simulink model "Intelligent_Vehicle"  (R2016a)
settings: Solver=FixedStepDiscrete  SolverMode=SingleTasking  StartTime=0.0  StopTime=350  FixedStep=1  RelTol=1e-3
libraries: simulink x1
settings Model: Creator=ihong-gyu  LastModifiedBy=Junghoon
settings DataIOCC: LimitDataPoints=on
settings OptimizationCC: DefaultParameterBehavior=Inlined  UseFloatMulNetSlope=on  InlineInvariantSignals=on  PassReuseOutputArgsAs=Individual arguments  ZeroExternalMemoryAtStartup=off  ZeroInternalMemoryAtStartup=off  NoFixptDivByZeroProtection=on  EfficientFloat2IntCast=on  OptimizeModelRefInitCode=on  LifeSpan=1
settings DebuggingCC: AllowSymbolicDim=off
settings HardwareCC: ProdBitPerPointer=32  ProdLargestAtomicFloat=None  ProdWordSize=32  ProdHWDeviceType=Infineon->TriCore
settings ModelReferenceCC: PropagateSignalLabelsOutOfModel=off
settings RTWCC: SystemTargetFile=ert.tlc  GenCodeOnly=on  TemplateMakefile=ert_default_tmf  GenerateReport=on  IncludeHyperlinkInReport=on  LaunchReport=on  GenerateTraceInfo=on  GenerateTraceReport=on  GenerateTraceReportSl=on  GenerateTraceReportSf=on  GenerateTraceReportEml=on  GenerateCodeMetricsReport=on
settings CodeAppCC: ForceParamTrailComments=on  IgnoreCustomStorageClasses=off  SimulinkDataObjDesc=on  CustomSymbolStrGlobalVar=rt$N$M  CustomSymbolStrType=$N$M  CustomSymbolStrFcn=$N$M$F  CustomSymbolStrMacro=$N$M  InsertBlockDesc=on
settings ERTTargetCC: GenerateSampleERTMain=on  IncludeMdlTerminateFcn=off  CombineSignalStateStructs=on  SupportNonFinite=off  InlinedParameterPlacement=NonHierarchical  ERTCustomFileTemplate=example_file_process.tlc  ERTFilePackagingFormat=CompactWithDataFile  PreserveExpressionOrder=on  PreserveIfCondition=on  ConvertIfToSwitch=off  SuppressUnreachableDefaultCases=off
settings ConfigurationSet: Description=SimMechanics 2G

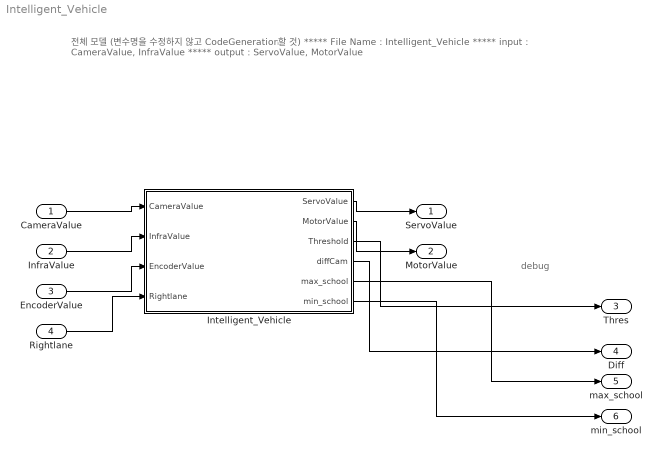
== system Intelligent_Vehicle ==
  note: debug
  note: 전체 모델
      | (변수명을 수정하지 않고 CodeGeneration할 것)
      |
      | ***** File Name : Intelligent_Vehicle
      | ***** input : CameraValue, InfraValue
      | ***** output : ServoValue, MotorValue
  CameraValue : Inport
  InfraValue : Inport  Port=2
  EncoderValue : Inport  Port=3
  Rightlane : Inport  Port=4
  "Intelligent_Vehicle " : Subsystem
      mask Display: image(imread('Images/self.jpeg'))
  ServoValue : Outport
  MotorValue : Outport  Port=2  OutDataTypeStr=int16
  Thres : Outport  Port=3
  Diff : Outport  Port=4
  max_school : Outport  Port=5
  min_school : Outport  Port=6
  wires:
  CameraValue/1 -> "Intelligent_Vehicle "/1(CameraValue)
  "Intelligent_Vehicle "/1(ServoValue) -> ServoValue/1
  "Intelligent_Vehicle "/2(MotorValue) -> MotorValue/1
  InfraValue/1 -> "Intelligent_Vehicle "/2(InfraValue)
  "Intelligent_Vehicle "/3(Threshold) -> Thres/1
  "Intelligent_Vehicle "/4(diffCam) -> Diff/1
  "Intelligent_Vehicle "/5(max_school) -> max_school/1
  "Intelligent_Vehicle "/6(min_school) -> min_school/1
  EncoderValue/1 -> "Intelligent_Vehicle "/3(EncoderValue)
  Rightlane/1 -> "Intelligent_Vehicle "/4(Rightlane)

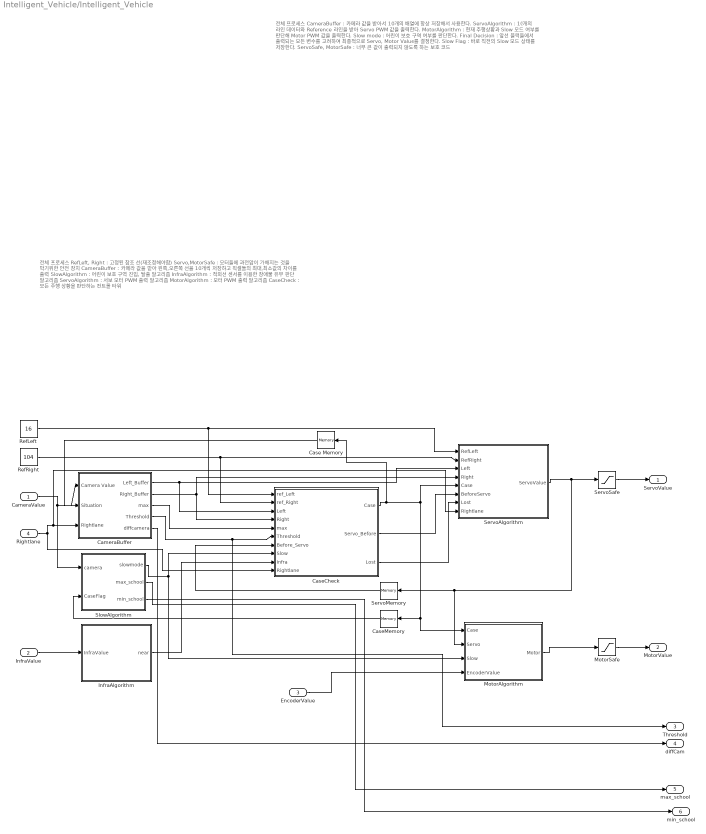
== system Intelligent_Vehicle/Intelligent_Vehicle  ==
  note: 전체 프로세스
      |
      | CameraBuffer : 카메라 값을 받아서 10개의 배열에 항상 저장해서 사용한다.
      | ServoAlgorithm : 10개의 라인 데이터와 Reference 라인을 받아 Servo PWM 값을 출력한다.
      | MotorAlgorithm : 현재 주행상황과 Slow 모드 여부를 판단해 Motor PWM 값을 출력한다.
      | Slow mode : 어린이 보호 구역 여부를 판단한다.
      | Final Decision : 앞선 블럭들에서 출력되는 모든 변수를 고려하여 최종적으로 Servo, Motor Value를 결정한다.
      | Slow Flag : 바로 직전의 Slow 모드 상태를 저장한다.
      | ServoSafe, MotorSafe : 너무 큰 값이 출력되지 않도록 하는 보호 코드
  note: 전체 프로세스
      |
      | RefLeft, Right : 고정된 참조 선(재조정해야함)
      | Servo,MotorSafe : 모터들에 과전압이 가해지는 것을 막기위한 안전 장치
      | CameraBuffer : 카메라 값을 받아 왼쪽,오른쪽 선을 10개씩 저장하고 픽셀들의 최대,최소값의 차이를 출력
      | SlowAlgorithm : 어린이 보호 구역 진입, 탈출 알고리즘
      | InfraAlgorithm : 적외선 센서를 이용한 장애물 유무 판단 알고리즘
      | ServoAlgorithm : 서보 모터 PWM 출력 알고리즘
      | MotorAlgorithm : 모터 PWM 출력 알고리즘
      | CaseCheck : 모든 주행 상황을 판단하는 컨트롤 타워
  CameraValue : Inport
  InfraValue : Inport  Port=2
  EncoderValue : Inport  Port=3
  Rightlane : Inport  Port=4
  CameraBuffer : Subsystem
      mask Display: image(imread('Images/linescan.jpg'))
  Case Memory : Memory  X0=1
  CaseCheck : MATLAB Function  TreatAsAtomicUnit=on
  CaseMemory : Memory
  InfraAlgorithm : MATLAB Function  TreatAsAtomicUnit=on
  MotorAlgorithm : Subsystem
      mask Display: image(imread('Images/dcmotor.jpeg'))
  MotorSafe : Saturate  UpperLimit=450  LowerLimit=-450
  RefLeft : Constant  Value=16  OutDataTypeStr=int16
  RefRight : Constant  Value=104  OutDataTypeStr=int16
  ServoAlgorithm : Subsystem
      mask Display: image(imread('Images/servo.jpg'))
  ServoMemory : Memory
  ServoSafe : Saturate  UpperLimit=100  LowerLimit=-100
  SlowAlgorithm : MATLAB Function  TreatAsAtomicUnit=on
  ServoValue : Outport
  MotorValue : Outport  Port=2  OutDataTypeStr=int16
  Threshold : Outport  Port=3
  diffCam : Outport  Port=4
  max_school : Outport  Port=5
  min_school : Outport  Port=6
  wires:
  CameraValue/1 -> CameraBuffer/1(Camera Value), SlowAlgorithm/1(camera)
  CaseCheck/1(Case) -> ServoAlgorithm/5(Case), MotorAlgorithm/1(Case), CaseMemory/1, Case Memory/1
  InfraValue/1 -> InfraAlgorithm/1(InfraValue)
  InfraAlgorithm/1(near) -> CaseCheck/9(Infra)
  ServoSafe/1 -> ServoValue/1
  MotorSafe/1 -> MotorValue/1
  CameraBuffer/3(max) -> CaseCheck/5(max)
  RefRight/1 -> ServoAlgorithm/2(RefRight), CaseCheck/2(ref_Right)
  RefLeft/1 -> ServoAlgorithm/1(RefLeft), CaseCheck/1(ref_Left)
  CameraBuffer/2(Right_Buffer) -> ServoAlgorithm/4(Right), CaseCheck/4(Right)
  CameraBuffer/1(Left_Buffer) -> ServoAlgorithm/3(Left), CaseCheck/3(Left)
  CaseCheck/2(Servo_Before) -> ServoAlgorithm/6(BeforeServo)
  ServoAlgorithm/1(ServoValue) -> MotorAlgorithm/2(Servo), ServoMemory/1, ServoSafe/1
  SlowAlgorithm/1(slowmode) -> CaseCheck/8(Slow), MotorAlgorithm/3(Slow)
  CaseMemory/1 -> SlowAlgorithm/2(CaseFlag)
  CaseCheck/3(Lost) -> ServoAlgorithm/7(Lost)
  ServoMemory/1 -> CaseCheck/7(Before_Servo)
  MotorAlgorithm/1(Motor) -> MotorSafe/1
  CameraBuffer/4(Threshold) -> Threshold/1, CaseCheck/6(Threshold)
  CameraBuffer/5(diffcamera) -> diffCam/1
  SlowAlgorithm/2(max_school) -> max_school/1
  SlowAlgorithm/3(min_school) -> min_school/1
  Case Memory/1 -> CameraBuffer/2(Situation)
  Rightlane/1 -> CaseCheck/10(Rightlane), ServoAlgorithm/8(Rightlane), CameraBuffer/3(Rightlane)
  EncoderValue/1 -> MotorAlgorithm/4(EncoderValue)

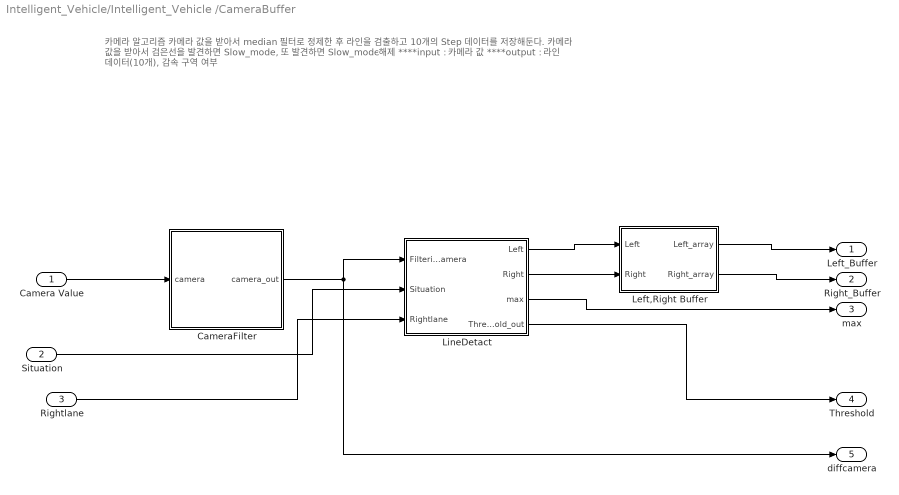
== system Intelligent_Vehicle/Intelligent_Vehicle /CameraBuffer ==
  note: 카메라 알고리즘
      |
      | 카메라 값을 받아서 median 필터로 정제한 후 라인을 검출하고 10개의 Step 데이터를 저장해둔다.
      | 카메라 값을 받아서 검은선을 발견하면 Slow_mode, 또 발견하면 Slow_mode해제
      |
      | ****input : 카메라 값
      | ****output : 라인 데이터(10개), 감속 구역 여부
  Camera Value : Inport  OutMin=[128]  OutMax=[128]  OutDataTypeStr=int16
  Situation : Inport  Port=2  OutMin=[128]  OutMax=[128]  OutDataTypeStr=int16
  Rightlane : Inport  Port=3  OutMin=[128]  OutMax=[128]  OutDataTypeStr=int16
  CameraFilter : MATLAB Function  TreatAsAtomicUnit=on
  Left,Right Buffer : MATLAB Function  TreatAsAtomicUnit=on
  LineDetact : MATLAB Function  TreatAsAtomicUnit=on
  Left_Buffer : Outport  OutMax=[10]  OutDataTypeStr=int16
  Right_Buffer : Outport  Port=2  OutMax=[10]  OutDataTypeStr=int16
  max : Outport  Port=3  OutMax=[10]  OutDataTypeStr=int16
  Threshold : Outport  Port=4  OutMax=[10]  OutDataTypeStr=int16
  diffcamera : Outport  Port=5  OutMax=[10]  OutDataTypeStr=int16
  wires:
  Left,Right Buffer/2(Right_array) -> Right_Buffer/1
  Left,Right Buffer/1(Left_array) -> Left_Buffer/1
  LineDetact/1(Left) -> Left,Right Buffer/1(Left)
  LineDetact/2(Right) -> Left,Right Buffer/2(Right)
  Camera Value/1 -> CameraFilter/1(camera)
  LineDetact/3(max) -> max/1
  CameraFilter/1(camera_out) -> diffcamera/1, LineDetact/1(Filtering_Camera)
  LineDetact/4(Threshold_out) -> Threshold/1
  Situation/1 -> LineDetact/2(Situation)
  Rightlane/1 -> LineDetact/3(Rightlane)

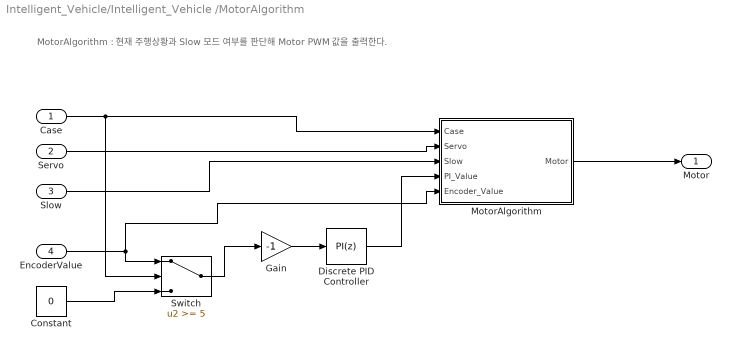
== system Intelligent_Vehicle/Intelligent_Vehicle /MotorAlgorithm ==
  note: MotorAlgorithm : 현재 주행상황과 Slow 모드 여부를 판단해 Motor PWM 값을 출력한다.
  Case : Inport  OutDataTypeStr=int16
  Servo : Inport  Port=2  OutDataTypeStr=int16
  Slow : Inport  Port=3  OutDataTypeStr=int16
  EncoderValue : Inport  Port=4  OutDataTypeStr=int16
  Constant : Constant  Value=0  OutDataTypeStr=int16
  Discrete PID Controller : simulink/Continuous/PID Controller  Controller=PI  TimeDomain=Discrete-time  SampleTime=1  IntegratorMethod=Forward Euler  FilterMethod=Forward Euler  Form=Parallel  UseFilter=on  ControllerParametersSource=internal  P=2.7  I=0.01  D=0  N=100  InitialConditionSource=internal  InitialConditionForIntegrator=0  InitialConditionForFilter=0  ExternalReset=none  ZeroCross=off  LimitOutput=on  UpperSaturationLimit=250  LowerSaturationLimit=-350  LinearizeAsGain=off  AntiWindupMode=none  Kb=1  TrackingMode=off  Kt=1  PParamMin=[]  PParamMax=[]  PParamDataTypeStr=double  IParamMin=[]  IParamMax=[]  IParamDataTypeStr=double  DParamMin=[]  DParamMax=[]  NParamMin=[]  NParamMax=[]  KbParamMin=[]  KbParamMax=[]  KtParamMin=[]  KtParamMax=[]  POutMin=[]  POutMax=[]  POutDataTypeStr=double  PGainOutDataTypeStr=double  PProdOutDataTypeStr=double  IOutMin=[]  IOutMax=[]  IOutDataTypeStr=double  IGainOutDataTypeStr=double  IProdOutDataTypeStr=double  DOutMin=[]  DOutMax=[]  NOutMin=[]  NOutMax=[]  KbOutMin=[]  KbOutMax=[]  KtOutMin=[]  KtOutMax=[]  IntegratorOutMin=[]  IntegratorOutMax=[]  IntegratorOutDataTypeStr=double  FilterOutMin=[]  FilterOutMax=[]  SumOutMin=[]  SumOutMax=[]  SumI1OutMin=[]  SumI1OutMax=[]  SumI2OutMin=[]  SumI2OutMax=[]  SumI3OutMin=[]  SumI3OutMax=[]  SumDOutMin=[]  SumDOutMax=[]  SaturationOutMin=[]  SaturationOutMax=[]  SaturationOutDataTypeStr=double  IntegratorContinuousStateAttributes=''  IntegratorStateMustResolveToSignalObject=off  IntegratorRTWStateStorageClass=Auto  FilterContinuousStateAttributes=''  FilterStateMustResolveToSignalObject=off  FilterRTWStateStorageClass=Auto  DifferentiatorICPrevScaledInput=0  DifferentiatorOutMin=[]  DifferentiatorOutMax=[]
  Gain : Gain  Gain=-1
  "MotorAlgorithm " : MATLAB Function  TreatAsAtomicUnit=on
  Switch : Switch  Threshold=5
  Motor : Outport  OutDataTypeStr=int16
  wires:
  Case/1 -> "MotorAlgorithm "/1(Case), Switch/2
  Servo/1 -> "MotorAlgorithm "/2(Servo)
  Slow/1 -> "MotorAlgorithm "/3(Slow)
  "MotorAlgorithm "/1(Motor) -> Motor/1
  Discrete PID Controller/1 -> "MotorAlgorithm "/4(PI_Value)
  Gain/1 -> Discrete PID Controller/1
  Switch/1 -> Gain/1
  Constant/1 -> Switch/3
  EncoderValue/1 -> Switch/1, "MotorAlgorithm "/5(Encoder_Value)

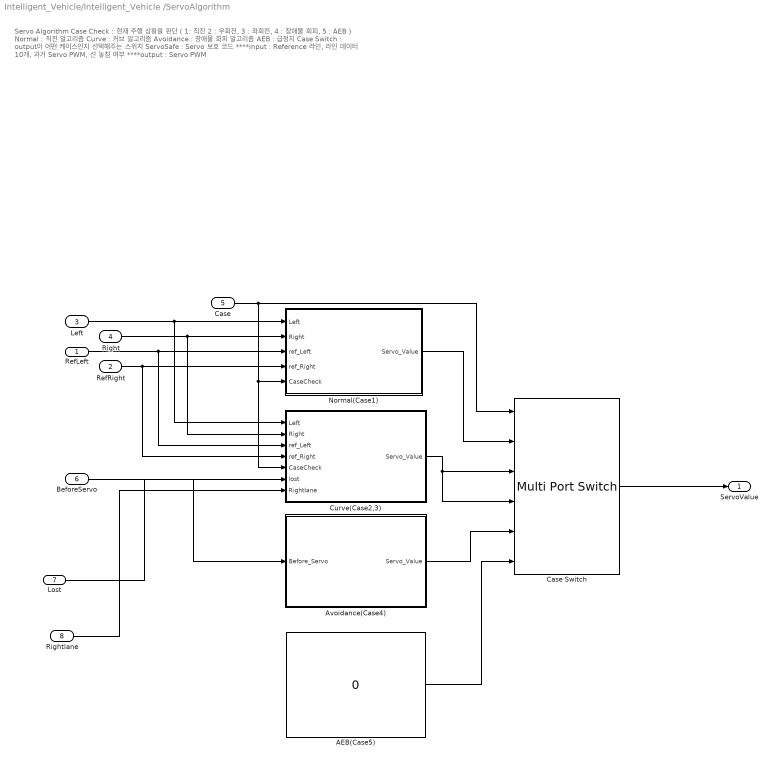
== system Intelligent_Vehicle/Intelligent_Vehicle /ServoAlgorithm ==
  note: Servo Algorithm
      |
      | Case Check : 현재 주행 상황을 판단 ( 1: 직진 2 : 우회전, 3 : 좌회전, 4 : 장애물 회피, 5 : AEB )
      | Normal : 직진 알고리즘
      | Curve : 커브 알고리즘
      | Avoidance : 장애물 회피 알고리즘
      | AEB : 급정지
      | Case Switch : output이 어떤 케이스인지 선택해주는 스위치
      | ServoSafe : Servo 보호 코드
      |
      | ****input : Reference 라인, 라인 데이터 10개, 과거 Servo PWM, 선 놓침 여부
      | ****output : Servo PWM
  RefLeft : Inport
  RefRight : Inport  Port=2
  Left : Inport  Port=3
  Right : Inport  Port=4
  Case : Inport  Port=5
  BeforeServo : Inport  Port=6
  Lost : Inport  Port=7
  Rightlane : Inport  Port=8
  AEB(Case5) : Constant  Value=0  OutDataTypeStr=int16
      mask Display: image(imread('Images/aeb.png'))
  Avoidance(Case4) : MATLAB Function  TreatAsAtomicUnit=on
  Case Switch : MultiPortSwitch  Inputs=5
      mask Display: image(imread('Images/switch.jpg'))
  Curve(Case2,3) : MATLAB Function  TreatAsAtomicUnit=on
  Normal(Case1) : MATLAB Function  TreatAsAtomicUnit=on
  ServoValue : Outport
  wires:
  Lost/1 -> Curve(Case2,3)/6(lost)
  Right/1 -> Curve(Case2,3)/2(Right), Normal(Case1)/2(Right)
  Case Switch/1 -> ServoValue/1
  RefRight/1 -> Curve(Case2,3)/4(ref_Right), Normal(Case1)/4(ref_Right)
  Curve(Case2,3)/1(Servo_Value) -> Case Switch/4, Case Switch/3
  BeforeServo/1 -> Avoidance(Case4)/1(Before_Servo)
  Normal(Case1)/1(Servo_Value) -> Case Switch/2
  Left/1 -> Curve(Case2,3)/1(Left), Normal(Case1)/1(Left)
  Case/1 -> Curve(Case2,3)/5(CaseCheck), Normal(Case1)/5(CaseCheck), Case Switch/1
  RefLeft/1 -> Curve(Case2,3)/3(ref_Left), Normal(Case1)/3(ref_Left)
  Avoidance(Case4)/1(Servo_Value) -> Case Switch/5
  AEB(Case5)/1 -> Case Switch/6
  Rightlane/1 -> Curve(Case2,3)/7(Rightlane)

== matlab function Intelligent_Vehicle/Intelligent_Vehicle /CameraBuffer/CameraFilter ==
  data: camera input int16 size=128; camera_out output int16 size=128
function camera_out= fcn(camera)

%%made by HongKyu 06.22
%%카메라 필터 모듈
%%카메라 값을 받아서 median 필터를 거친 후 차분값을 저장한다

%%전역 변수 초기화
persistent  lastpixel;
persistent  diff_camera;



if isempty(lastpixel)
    lastpixel=int16(1500);
end
if isempty(diff_camera)
    diff_camera = camera;
end



%%지역 변수 초기화
camera_out = camera;


%% 끝값들을 필터 적용(3,4개씩) 


%% 중간값들을 필터 적용 (5개씩)


%% 차분을 저장 
for i=2:128
    
    diff_camera(i)=camera(i)-lastpixel;
    camera_out(i)=diff_camera(i);
    lastpixel=camera(i-1);
end

== matlab function Intelligent_Vehicle/Intelligent_Vehicle /CameraBuffer/LineDetact ==
  data: Filtering_Camera input int16 size=128; Left output int16 size=1; Right output int16 size=1; max output; Threshold_out output; Situation input; Rightlane input
function [Left,Right,max,Threshold_out] = fcn(Filtering_Camera,Situation, Rightlane)

%%made by HongKyu 06.22
%%라인 검출 모듈
%%필터링 된 카메라 차분 값 중에서 변화의 최대값을 선으로 인식한다
%%최소값을 저장하는 이유는 SLOW 모드를 받아들일 때 사용하려 했으나 우꿍1 알고리즘을 참고하여 사용안할 예정 
%%알고리즘 by 우꿍2

%%전역 변수 초기화 
persistent maxmindiff;
persistent LPF_initcount;
persistent  array_max;
persistent  sum_max;
persistent Threshold;

if isempty(maxmindiff)
    maxmindiff = 0;
end
if isempty(LPF_initcount)
    LPF_initcount = 0;
end
if isempty(array_max)
   array_max = int16(zeros(1,10));
end
if isempty(sum_max)
   sum_max = int16(0);
end
if isempty(Threshold)
   Threshold = int16(0);
end


%%지역 변수 초기화
%%아예 값이 안들어오는걸 보기위해 Right는 125, Left는 2로
Right = int16(125);
Left = int16(4);
sum = int16(0);
max = Filtering_Camera(3);
min = Filtering_Camera(3);

L_missflag = int16(0);
R_missflag = int16(0);
%%차분의 합과 최대값,최소값 위치를 저장 
for i=4:125
    sum=sum+abs(Filtering_Camera(i));
    if Filtering_Camera(i)>max
        max = Filtering_Camera(i);
    end
    if Filtering_Camera(i)<min
        min = Filtering_Camera(i);
    end
    
end

%%픽셀 최대값과 최소값의 차이를 얻음 (차선을 못보고 흰선만 볼 때를 위한 변수)

%% Threshold에 LPF (일단 보류)
% if(LPF_initcount <10)
% sum_max = sum_max + max;
%     if(LPF_initcount==9)
%         sum_max = sum_max/9;
%     end
% LPF_initcount = LPF_initcount+1;
% Threshold=fix(max/2);

% else
% Threshold=fix((((0.4*max)+(0.6*sum_max))/2));
% sum_max=fix((0.4*max)+(0.6*sum_max));

% end

%% 최대값을 이용한 임계값 설정 

% Threshold = fix((sum/122+max)/3);
% if Threshold < int16(750)
%   Threshold = int16(750);
% end

Threshold = max/2;
if Threshold < int16(700)
    Threshold = int16(700);
end


%% 임계값을 넘는 최대값을 다시 한번 확인( 확인 코드 ) 
for i=4:62
    if Threshold < Filtering_Camera(i)
        if Filtering_Camera(i)>Filtering_Camera(Left)
        Left=int16(i-2);
        L_missflag=L_missflag+1;
        end
    end
end

for j=61:125
    if -Threshold > Filtering_Camera(186-j)
        if Filtering_Camera(186-j) < Filtering_Camera(Right)
        Right=int16(186-j);
        R_missflag=R_missflag+1;
        end
    end
end

if L_missflag == 0
    Left = int16(1);
end

if R_missflag == 0
    Right = int16(127);
end

if Situation == 3 && Right == 127 && Rightlane == 1
        Right = Left;
        Left = int16(1);
end

if Situation == 3 && Right == 127 && Rightlane == 0
    Left = Right;
    Right = int16(127);
end

if Situation == 2 && Left == 1 && Rightlane == 1
    Left = Right;
    Right = int16(127);
end

if Situation == 2 && Left == 1 && Rightlane == 0
        Right = Left;
        Left = int16(1);
end
    
Threshold_out =Threshold;

== matlab function Intelligent_Vehicle/Intelligent_Vehicle /ServoAlgorithm/Avoidance(Case4) ==
  data: Before_Servo input int16 size=1; Servo_Value output int16 size=1
function Servo_Value  = fcn(Before_Servo)

%%made by HongKyu 06.22
%%장애물 회피 알고리즘
%%장애물 회피 by 연규환

%%Case Check에서 넘어온 서보값을 출력 
Servo_Value = Before_Servo;

== matlab function Intelligent_Vehicle/Intelligent_Vehicle /MotorAlgorithm/MotorAlgorithm  ==
  data: Case input int16; Motor output int16; Servo input int16; Slow input int16; PI_Value input; Encoder_Value input
function Motor  = fcn(Case,Servo,Slow, PI_Value, Encoder_Value)

persistent Case2_BrakeFlag;
if isempty(Case2_BrakeFlag)
   Case2_BrakeFlag = int16(0);
end

persistent AEB_revFlag;
if isempty(AEB_revFlag)
   AEB_revFlag = int16(0);
end

%%made by HongKyu 06.22
%%모터 PWM 값
%%조향값에 따라서 모터값을 선형적으로 변경 ( 부드럽게 커브를 돌 수 있다)


%% 전체 케이스 분류
    %%AEB일 때 
if  Case == 5

    if AEB_revFlag == int16(0);
        if Encoder_Value>10
            Motor = int16(-250);
            AEB_revFlag = int16(1);
        else
        Motor = int16(PI_Value);
        end
    else
    Motor = int16(PI_Value);
    Case2_BrakeFlag = int16(0);
    end
    %%SlowMode 일 때
elseif Slow==1
    Motor = int16(50);
    Case2_BrakeFlag = int16(0);
    %%평상시
elseif Case == 1
    Motor = int16(200-abs(1*Servo));
    Case2_BrakeFlag = int16(0);
    
elseif Case == 2
    if Encoder_Value>20 && Case2_BrakeFlag == int16(0)
        Motor = int16(-200);
        Case2_BrakeFlag = int16(1);
    else
    Motor = int16(100);
    end
    
else
    Motor = int16(120);
    Case2_BrakeFlag = int16(0);
end

== matlab function Intelligent_Vehicle/Intelligent_Vehicle /InfraAlgorithm ==
  data: InfraValue input int16; near output int16
function near = fcn(InfraValue)

%%made by HongKyu 06.22
%%적외선 센서 모듈
%%적외선 센서를 이용해 근접한 물체 여부 파악

%%전역 변수 선언
persistent  Infra_Count;
if isempty(Infra_Count)
   Infra_Count = 0;
end

%%값이 400이 넘으면 카운트를 올리고 3개 이상 들어오면 가깝다고 판단. 
if InfraValue>350
    Infra_Count=Infra_Count+1;
else
    Infra_Count=0;
end

if Infra_Count>2
    near=int16(1);
else
    near=int16(0);
end

== matlab function Intelligent_Vehicle/Intelligent_Vehicle /CameraBuffer/Left,Right Buffer ==
  data: Left input int16 size=1; Left_array output int16 size=[1 10]; Right input int16 size=1; Right_array output int16 size=[1 10]
    function [Left_array,Right_array] = fcn(Left,Right)

%%made by HongKyu 06.22
%%라인 검출 저장소(Buffer) 
%%왼쪽 오른쪽 선에 대한 정보를 10개 저장해둔다.
%%지금은 커브를 도는데 일부분 사용하지만 확장해서 더 사용하면 좋음 

%%전역 변수 초기화 
persistent  array_left;
persistent  array_right;

if isempty(array_left)
   array_left = int16(zeros(1,10));
end

if isempty(array_right)
   array_right = int16(zeros(1,10));
end


%%10개의 변수를 저장하는 배열을 갱신하고 출력 
for i=0:8
    array_left(10-i)=array_left(9-i);
    array_right(10-i)=array_right(9-i);
end

array_left(1)=Left;
array_right(1)=Right;

Left_array=array_left;
Right_array=array_right;

== matlab function Intelligent_Vehicle/Intelligent_Vehicle /SlowAlgorithm ==
  data: camera input int16 size=128; slowmode output int16 size=1; CaseFlag input; max_school output; min_school output




function [slowmode, max_school, min_school]  = fcn(camera, CaseFlag)

%%made by HongKyu 06.22
%%어린이 보호 구역 모듈
%%카메라 값의 변화를 이용해서 파악

%%전역 변수 초기화
persistent  slow_filter;
persistent  slow_now;
persistent  change_one;
persistent  camera_before;
persistent  schoolzonesum;
persistent schoolzonevalue;
persistent startcount;

if isempty(slow_filter)
    slow_filter = int16(0);
end

if isempty(slow_now)
    slow_now = int16(0);
end

if isempty(change_one)
    change_one = 0;
end

if isempty(camera_before)
    camera_before = camera;
end


if isempty(schoolzonesum)
    schoolzonesum = int16(zeros(1,3));
end

if isempty(schoolzonevalue)
    schoolzonevalue = int16(0);
end


if isempty(startcount)
    startcount = int16(0);
end

schoolzonesum(1)=int16(0);

for j=30:98
    schoolzonesum(1) = schoolzonesum(1) + camera(j)/69;
end
for i=0:1
    schoolzonesum(3-i)=schoolzonesum(2-i);
end

max_school = max([schoolzonesum(3) schoolzonesum(2) schoolzonesum(1)]);
min_school = min([schoolzonesum(3) schoolzonesum(2) schoolzonesum(1)]);

if startcount > 300
    if CaseFlag ~= 4
        
        %%schoolzonesum(2)는 이전 카메라 합 (1)은 현재 카메라 합
        schoolzonevalue = int16((max_school-min_school)*100/max_school);
        %%밝기 변화가 15퍼센트 이상
        if schoolzonevalue > 50
            %%school1 --> by school2 --> cy q0 = by/cy
            %%slow_now flag 0 --> 1
            if(slow_now == int16(0))
                slow_now = int16(1);
                
                %%slow_now flag 1 --> 0
            else
                slow_now = int16(0);
            end
            %%카운터 초기화
            startcount = int16(0);
        end
    end
    
end
%%스쿨존 못잡으면
if startcount<2000
    startcount = startcount + 1 ;
end




%%출력 : SLOWMODE = 1; 어린이 보호구역, SLOWMODE = 0; 일반 구역
slowmode=slow_now;

== matlab function Intelligent_Vehicle/Intelligent_Vehicle /CaseCheck ==
  data: ref_Left input; ref_Right input; Left input int16 size=[1 10]; Case output int16 size=1; Right input int16 size=[1 10]; max input; Threshold input; Before_Servo input; Servo_Before output int16 size=1; Slow input; Infra input; Lost output; Rightlane input

function [Case,Servo_Before,Lost]  = fcn(ref_Left, ref_Right,Left, Right, max,Threshold, Before_Servo,Slow,Infra, Rightlane)

%%made by HongKyu 06.22
%%Case 분류 알고리즘
%%상황 판단을 하고 어떤 주행 상황인지를 출력

%% Case 1 = 보통 주행
%% Case 2 = 우회전
%% Case 3 = 좌회전
%% Case 4 = 장애물 회피
%% Case 5 = AEB

%%전역 변수 초기화
persistent Situation;
persistent Servo_store;
persistent Curve_Flag;
persistent Big_Change;
persistent line;
persistent locationcount;
persistent secondlocationcount;
persistent thirdlocationcount;
persistent Avoidancecount;


if isempty(Situation)
    Situation = 1;
end
if isempty(Servo_store)
    Servo_store = int16(0);
end
if isempty(Curve_Flag)
    Curve_Flag = 0;
end
if isempty(Big_Change)
    Big_Change=0;
end

if isempty(line)
    line=0;
end

if isempty(locationcount)
    locationcount = 0;
end
if isempty(secondlocationcount)
    secondlocationcount = 0;
end
if isempty(thirdlocationcount)
    thirdlocationcount = 0;
end
if isempty(Avoidancecount)
    Avoidancecount = 0;
end


lost=0;



%%가장 먼저 적외선 센서 인식이 되었는지 확인한다. 장애물 회피 혹은 AEB 상황을 판단.
if Infra == 1
    if Slow == 1
        Situation = 4;
    else
        Situation = 5;
    end
    %%장애물이 없는 일반 상황에서의 알고리즘
    
    %%Infra 값이 없고(0)
else
    
    if Slow==0
        if line==1
            Situation = 4;
        end
    end
    
    %%장애물 회피 중일 때는 직진, 회전등을 판단하지 않는다
    %%장애물 회피 중이 아니라면,
    if Situation ~=4
        
        %%카메라 값을 받았을 때 최대값과 최소값 차이가 Threshold이상 나지 않으면 흰색 부분만 보는 것으로 간주해서 선을 놓쳤다고 판단
        if max<Threshold
            %%선을 놓침
            lost=1;
        else
            %%선을 놓치지 않음
            lost=0;
        end
        
        
        %%선을 놓쳤다면 회전하던 상황을 그대로 유지한다. MAXMIN을 정상적으로 받을 때 까지
        if lost == 0
            %%직진 상태였으면
            if Situation==1
                %%과거 서보 정보를 저장해둔다. 직진을 벗어나는 순간 필요하기 때문에 계속 저장해둔다.
                %%나중에 최적화하면 그냥 회전 시에 값으로 넣어줘도 될 것 같다.
                Servo_store = Before_Servo;
                
                %%처음에 버퍼값이 없을 때는 회전을 판별하지 않는다.
                
                %%좌측,우측의 라인이 한번에 40 픽셀 이상 움직이거나(확바뀔때)
                %%좌우측 선 차이가 20이하로 날 때(바뀌다가 중간에 걸칠때)
                
                %% 우측 차선에서의 코너 진입 판단
                if (Left(1)-Left(2))>40 && Rightlane == 1
                    Situation = 3;
                end
                
                if (Left(2)-Left(1))>40 && Rightlane == 1
                    Situation = 2;
                end
                
                %% 좌측 차선에서의 코너 진입 판단
                if (Left(1)-Left(2))>40 && Rightlane == 0
                    Situation = 2;
                end
                
                
                if (Left(2)-Left(1))>40 && Rightlane == 0
                    Situation = 3;
                end
                
            end
        end
        
        %%회전 중에 탈출 조건
        if Situation==2
            %%Reference 라인과의 차이가 15 이하로 나는 순간을 잡아낸다.
            if abs(Left(1)-ref_Left)<=15 && abs(Right(1)-ref_Right)<=15
                %%2번 이상들어오면 탈출한다
                Curve_Flag=Curve_Flag+1;
            else
                Curve_Flag=0;
            end
            
            
            %%2번 이상들어오면 탈출한다
            if Curve_Flag>1
                Situation=1;
                Curve_Flag=0;
            end
        end
        
        if Situation==3
            %%Reference 라인과의 차이가 15 이하로 나는 순간을 잡아낸다.
            if abs(Left(1)-ref_Left)<=15 && abs(Right(1)-ref_Right)<=15
                %%2번 이상들어오면 탈출한다
                Curve_Flag=Curve_Flag+1;
            else
                Curve_Flag=0;
            end
            
            %%2번 이상들어오면 탈출한다
            if Curve_Flag>1
                Situation=1;
                Curve_Flag=0;
            end
            
        end
        
    end
end



%% 장애물 회피 알고리즘
if Situation==4
    %%회전할 때 사용하던 Servo_Before 값에 조향값을 넣어서 전달할 것이다
    %%장애물 회피 시에만 이렇게 사용
    %%뒷부분에서 CaseCheck에 관여하는 것을 막기위한 방법
    if Slow == 0 && Rightlane == 1
         Servo_store = int16(-20);
         if Avoidancecount < 100
             Avoidancecount = Avoidancecount + 1;
         else
             Servo_store = int16(10);
             if abs(Left(1)-ref_Left)<=20 && abs(Right(1)-ref_Right)<=20
                 Avoidancecount = 0;
                 line = 0;
                Situation=1;
             end
         end
         
    elseif Slow == 0 && Rightlane == 0
         Servo_store = int16(20);
         if Avoidancecount < 100
             Avoidancecount = Avoidancecount + 1;
         else
             Servo_store = int16(-10);
             if abs(Left(1)-ref_Left)<=20 && abs(Right(1)-ref_Right)<=20
                 Avoidancecount = 0;
                 line = 0;
                Situation=1;
             end
         end
        
    elseif ( line==0 && Rightlane == 1 ) || ( line==1 && Rightlane == 0 ) %% 오른쪽 차선에서 장애물만날시
        Servo_store = int16(100);
        
        %%왼쪽 차선이 안보일때
        if Left(1) == 1 
            Servo_store = int16(50);
            locationcount = 1;
        end
        if locationcount ==1
            Servo_store = int16(0);
            %%왼쪽차선을 찾으면 탈출
            if (20 < Left(1) && Left(1) < 51)
                locationcount = 0;
                line = mod(line+1,2);
                Situation=1;
            end
        end
        
    elseif ( line==1 && Rightlane == 1 ) || ( line==0 && Rightlane == 0 )  %%왼쪽 차선에서 진입
        Servo_store = int16(-100);
        
        if Right(1)==127  %% 오른쪽 차선이 안보일때
            locationcount = 1;
            Servo_store = int16(-50);
        end
        if locationcount ==1
            Servo_store = int16(0);
            %%오른 쪽 차선을 찾으면 탈출
            if (80 < Right(1) && Right(1) < 120)
                locationcount = 0;
                line = mod(line+1,2);
                Situation=1;
            end
        end
    end
end

%%AEB 탈출
if Situation == 5
    if Infra == 0
        Situation = 1;
    end
end


%%출력 : 과거 서보값, 주행 케이스, 선을 놓쳤을 때 케이스
Servo_Before = Servo_store;
Case = int16(Situation);
Lost = int16(lost);

== matlab function Intelligent_Vehicle/Intelligent_Vehicle /ServoAlgorithm/Curve(Case2,3) ==
  data: Left input int16 size=10; Servo_Value output int16 size=1; Right input int16 size=10; ref_Left input; ref_Right input; CaseCheck input int16 size=1; lost input; Rightlane input
function Servo_Value  = fcn(Left,Right,ref_Left,ref_Right,CaseCheck,lost, Rightlane)

%%made by HongKyu 06.22
%%커브 조향 값 
%%우회전 좌회전에 대한 조향 PWM 값을 출력 


%%전역 변수 초기화 
persistent Case2_PGain;
persistent Case2_PGainwell;

persistent Case3_PGain;
persistent Case3_PGainwell;

if isempty(Case2_PGain)
    Case2_PGain = 2.5;
end

if isempty(Case2_PGainwell)
    Case2_PGainwell = 3;
end

if isempty(Case3_PGain)
    Case3_PGain = 1.5;
end

if isempty(Case3_PGainwell)
    Case3_PGainwell = 1.5;
end

Servo_Value = int16(0);

  errorR = ref_Right-Right(1);
  errorL = ref_Left-Left(1);


%%우회전인지 좌회전인지 판단하고 값을 넣는다. 
if CaseCheck==2
    %%차선을 놓친 상황에서는 현재 회전 방향으로 최고 조향을 넣어준다. 
    if lost==1
        if Rightlane == 1
            Servo_Value = int16(-100);
        elseif Rightlane == 0
            Servo_Value = int16(100);
        end
    
    %%차선을 잘 찾아서 따라갈 때는 회전 상황으로 들어가는 순간의 조향값에 에러값을 P 제어값을 더해서 넣어준다. 
    else
        if Left(1)>60 && Rightlane == 1
            Servo_Value = int16(Case2_PGain*errorL);
        elseif Right(1)<61 && Rightlane == 0
            Servo_Value = int16(Case2_PGain*errorR);
        else
            Servo_Value=Case2_PGainwell*(errorR + errorL)/2;
        end
    end
    
elseif CaseCheck==3
     %%차선을 놓친 상황에서는 현재 회전 방향으로 최고 조향을 넣어준다. 
    if lost==1
        if Rightlane == 1
            Servo_Value = int16(100);
        elseif Rightlane == 0
            Servo_Value = int16(-100);
        end
         
        %%차선을 잘 찾아서 따라갈 때는 회전 상황으로 들어가는 순간의 조향값에 에러값을 P 제어값을 더해서 넣어준다.
    else
        if Right(1)<61 && Rightlane == 1
            Servo_Value = int16(Case3_PGain*errorR);
        elseif Left(1)>60 && Rightlane == 0
            Servo_Value = int16(Case3_PGain*errorL);
        else
            Servo_Value=Case3_PGainwell*(errorR + errorL)/2;
        end
    end
    
end

== matlab function Intelligent_Vehicle/Intelligent_Vehicle /ServoAlgorithm/Normal(Case1) ==
  data: Left input int16 size=[1 10]; Servo_Value output int16 size=1; Right input int16 size=[1 10]; ref_Left input int16 size=1; ref_Right input int16 size=1; CaseCheck input int16 size=1
function Servo_Value = fcn( Left,Right, ref_Left, ref_Right,CaseCheck)


%%made by HongKyu 06.22
%%06.29 수정 by 정훈
%%직진 서보 값 
%%케이스 값과 선 정보를 받아서 조향 PWM 값을 출력한다.

%%전역 변수 초기화 - 좌 우측 서보 P 게인 값(PD 제어를 할 것이므로 알고리즘과 변수 추가할 예정)

persistent Case1_Pgain_1Left;
persistent Case1_Pgain_2Left;
persistent Case1_Pgain_3Left;
persistent Case1_Pgain_4Left;
persistent Case1_Pgain_5Left;

persistent Case1_Pgain_1Right;
persistent Case1_Pgain_2Right;
persistent Case1_Pgain_3Right;
persistent Case1_Pgain_4Right;
persistent Case1_Pgain_5Right;


if isempty(Case1_Pgain_1Left)
    Case1_Pgain_1Left = 1;
end
if isempty(Case1_Pgain_2Left)
    Case1_Pgain_2Left = 1.2;
end
if isempty(Case1_Pgain_3Left)
    Case1_Pgain_3Left = 1.4;
end
if isempty(Case1_Pgain_4Left)
    Case1_Pgain_4Left = 2;
end
if isempty(Case1_Pgain_5Left)
    Case1_Pgain_5Left = 2.2;
end

if isempty(Case1_Pgain_1Right)
    Case1_Pgain_1Right = 1;
end
if isempty(Case1_Pgain_2Right)
    Case1_Pgain_2Right = 1.2;
end
if isempty(Case1_Pgain_3Right)
    Case1_Pgain_3Right = 1.4;
end
if isempty(Case1_Pgain_4Right)
    Case1_Pgain_4Right = 2;
end
if isempty(Case1_Pgain_5Right)
    Case1_Pgain_5Right = 2.2;
end
%%지역 변수 초기화 
Servo_P = int16(0);
Servo_LP = int16(0);
Servo_RP = int16(0);

%%직진 상황인지 검증 - 만약 아니라면 계산 없이 그냥 0 값을 내뱉는다. 
if CaseCheck==1
    
    %%좌,우측 에러
    %%우로 가야하면 eL, eR이 양수겠지 좌는 음수
    
    errorL = ref_Left - Left(1);
    errorR = ref_Right - Right(1);
    
    
    if abs(errorL)<7
        Servo_LP = Case1_Pgain_1Left*errorL;
        
    elseif abs(errorL)>=7 && abs(errorL)<16
        Servo_LP = Case1_Pgain_2Left*errorL;
        
    elseif abs(errorL)>=16 && abs(errorL)<22
        Servo_LP = Case1_Pgain_3Left*errorL;
        
    elseif abs(errorL)>=22 && abs(errorL)<29
        Servo_LP = Case1_Pgain_4Left*errorL;
        
    elseif abs(errorL)>=29
        Servo_LP = Case1_Pgain_5Left*errorL;
    end
    
    if abs(errorR)<8
        Servo_RP = Case1_Pgain_1Right*errorR;
        
    elseif abs(errorR)>=8 && abs(errorR)<18
        Servo_RP = Case1_Pgain_2Right*errorR;
        
    elseif abs(errorR)>=18 && abs(errorR)<24
        Servo_RP = Case1_Pgain_3Right*errorR;
        
    elseif abs(errorR)>=24 && abs(errorR)<34
        Servo_RP = Case1_Pgain_4Right*errorR;
        
    elseif abs(errorR)>=34
        Servo_RP = Case1_Pgain_5Right*errorR;
    end
   %%서보값은 -100이 최우측, 100이 최좌측이다 고로 부호가 반대로 되어야함  
   Servo_P = (Servo_RP+Servo_LP)/2;
end



%%출력 : 조향 PWM 
Servo_Value = int16(Servo_P);
